simulink model "power_brushlessDCmotor_moog2328_control_scheme"  (R2022a)
settings: Solver=ode4  StartTime=0  StopTime=2  FixedStep=Ts  MaxStep=1e-6  RelTol=1e-6  AbsTol=1e-6  EnableMultiTasking=on
PreLoadFcn:
  | assignin('base','Ts',[5e-6])
values from neighbouring files (symbols this model uses):
  F = 49.387e-4*2/1000    (= 9.8774e-06)    [power_brushlessDCmotor_moog2328_control_scheme.m]
  J = 465.8e-7    (= 4.658e-05)    [power_brushlessDCmotor_moog2328_control_scheme.m]
  La = 0.17e-3    (= 0.00017)    [power_brushlessDCmotor_moog2328_control_scheme.m]
  Lb = 0.17e-3    (= 0.00017)    [power_brushlessDCmotor_moog2328_control_scheme.m]
  Lc = 0.17e-3    (= 0.00017)    [power_brushlessDCmotor_moog2328_control_scheme.m]
  N = 297.5    [power_brushlessDCmotor_moog2328_control_scheme.m]
  p = 4    [power_brushlessDCmotor_moog2328_control_scheme.m]
  Ra = 0.1    [power_brushlessDCmotor_moog2328_control_scheme.m]
  Rb = 0.1    [power_brushlessDCmotor_moog2328_control_scheme.m]
  Rc = 0.1    [power_brushlessDCmotor_moog2328_control_scheme.m]
  trap = sin((pi-Flat/180*pi)/2)    [power_brushlessDCmotor_moog2328_control_scheme.m]
  Ts = 5e-5    (= 5e-05)    [power_brushlessDCmotor_moog2328_control_scheme.m]
undefined symbols (not defined in the file or in its folder): DiscIntNeverNeededParam, find_system, sgn
libraries: simulink x7, spsDiodeLib x6, spsMosfetLib x6, spsCurrentMeasurementLib x4, spsVoltageMeasurementLib x4, spsParallelRLCBranchLib x3, spsGroundLib x3, spsControlledVoltageSourceLib x3, spsSeriesRLCBranchLib x3, simulink_extras x3, spsDCVoltageSourceLib x1, spspowerguiLib x1
Description:
  | This demonstration illustrates use of the BLDC in a closed-loop
  | speed and voltage control on a 1 kW, 3000 rpm industrial motor
settings Model: Creator=Olivier Tremblay  LastModifiedBy=marin
settings SolverCC: AutoScaleAbsTol=off  AlgebraicLoopSolver=TrustRegion
settings DataIOCC: LimitDataPoints=on  SaveFormat=Array  SignalLoggingSaveFormat=ModelDataLogs  ReturnWorkspaceOutputs=off  SignalLoggingName=sigsOut
settings OptimizationCC: ExpressionDepthLimit=2147483647  InitFltsAndDblsToZero=on  LifeSpan=inf
settings DebuggingCC: SaveWithParameterizedLinksMsg=none  UnderspecifiedInitializationDetection=Classic  MergeDetectMultiDrivingBlocksExec=none  SignalResolutionControl=TryResolveAllWithWarning  MultiTaskDSMMsg=warning  MultiTaskCondExecSysMsg=none  SigSpecEnsureSampleTimeMsg=none  FcnCallInpInsideContextMsg=warning  UnconnectedInputMsg=warning  UnconnectedOutputMsg=warning  UnconnectedLineMsg=warning  StateNameClashWarn=warning  SFUnexpectedBacktrackingDiag=warning  SFNoUnconditionalDefaultTransitionDiag=warning  SFExecutionAtInitializationDiag=none  SFMachineParentedDataDiag=warning  ArithmeticOperatorsInVariantConditions=warning
settings HardwareCC: ProdBitPerPointer=32  ProdBitPerSizeT=32  ProdBitPerPtrDiffT=32  ProdLargestAtomicFloat=None  ProdIntDivRoundTo=Undefined  ProdEndianess=Unspecified  ProdWordSize=32  ProdHWDeviceType=32-bit Generic  TargetUnknown=on
settings ModelReferenceCC: PropagateSignalLabelsOutOfModel=off
settings SFSimCC: SimUseLocalCustomCode=off  CustomCodeUndefinedFunction=UseInterfaceOnly
settings RTWCC: RTWUseLocalCustomCode=off  DLArmComputeVersion=19.05
settings CodeAppCC: StateflowObjectComments=on
settings GRTTargetCC: TargetFcnLib=ansi_tfl_tmw.mat  TargetLangStandard=C89/C90 (ANSI)  CombineOutputUpdateFcns=off  GRTInterface=on
settings ConfigComp: CovMetricSettings=dw  CovSaveCumulativeToWorkspaceVar=on  CovSaveSingleToWorkspaceVar=on  CovExternalEMLEnable=off
settings SimscapeCC: SimscapeNormalizeSystem=off

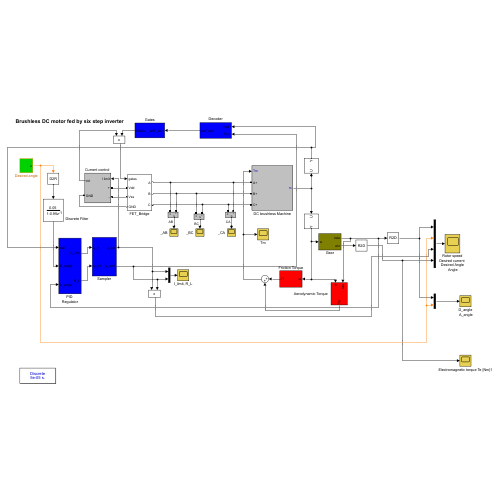
[thumbnail: Simulink's stored preview of the top-level diagram]
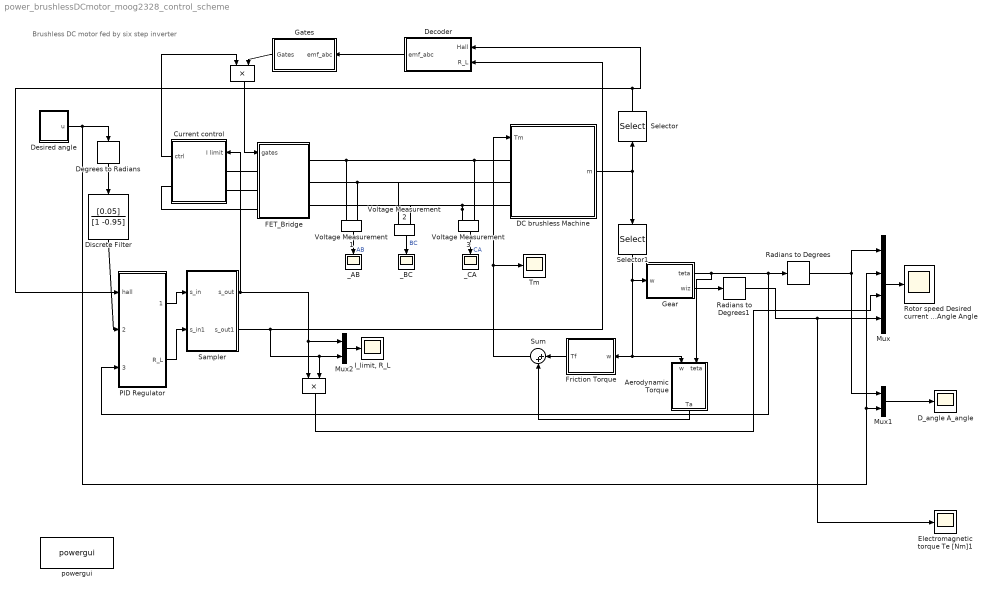
== system power_brushlessDCmotor_moog2328_control_scheme ==
  note: Brushless DC motor fed by six step inverter
  " " : Product  RndMeth=Zero
  " " : Product  RndMeth=Zero
  " Discrete Filter" : DiscreteFilter  Numerator=[0.05]  Denominator=[1 -0.95]  SampleTime=Ts
  " Current control " : Subsystem  mask(Current control){R=0.02, R1=0.01, C=4700e-6, V1=14.31/100, V=28}
      mask prompts: R "Resistance R [ohm]"; R1 "Resistance R1 [ohm]"; C "Capacitance C [F]"; V1 "Control voltage [V]"; V "DC source [V]"
  "Aerodynamic Torque " : Subsystem  mask(Aerodynamic Torque and friction){Ta=100, G=N, eta=0.7, Tgv=0, Tgf=0}
      mask prompts: Ta "Aerodinamic Torque [Nm]"; G "Gear coeficient"; eta "Eficiency"; Tgv "Fg viscous friction"; Tgf "Kgf columb friction"
  DC brushless Machine : Subsystem  AncestorBlock=powerlib/Machines/DC Machine  LoadFcn=find_system(gcs,'FollowLinks', 'on', 'LookUnderMasks', 'all');
      settings: OpenFcn=power_openblockproxy();
  D_angle A_angle : Scope
  Decoder : Subsystem  mask(Decoder){}
      mask help:
      | Hal
      | 	to	emf_abc
      | R or L
  Degrees to Radians : simulink_extras/Transformations/Degrees to Radians
  "Desired angle " : Subsystem  mask(Deaired angle){Fo=1, f=2.5, of=6, ch=1, an=-1}
      mask prompts: Fo "Desired angle [deg]"; f "Freqency [Hz]"; of "ofs"; ch "1 for sin(x), -1 for square(x)"; an "1 for angle meas. -1 for simul."
      mask init:
      | Fid=Fo
  Electromagnetic torque Te [Nm]1 : Scope
  FET_Bridge : Subsystem
  Friction Torque : Subsystem  mask(Friction Torque){Tf=0.303*0.05}
      mask prompts: Tf "Friction Torque [Nm]"
  Gates : Subsystem  mask(Gates){}
      mask help: Convert emf_abc in to signal for gates
  Gear : Subsystem  mask(Gear){}
      mask help: Integration and gear reduction
  "I_limit, R_L" : Scope
  Mux : Mux
  Mux1 : Mux  Inputs=2
  Mux2 : Mux  Inputs=2
  PID Regulator : Subsystem  mask(PID Regulator){KI=27.0082733381866, KP=1.97984715541991*65, KD=0.0105535523473669*35, Ao=10, Inom=14.31, Boost=1}
      mask prompts: KI "Integral gain"; KP "Proportional gain"; KD "Differential gain"; Ao "Ao gain"; Inom "Nominal current [A]"
  Radians to Degrees : simulink_extras/Transformations/Radians to Degrees
  Radians to Degrees1 : simulink_extras/Transformations/Radians to Degrees
  Rotor speed Desired current Desired Angle Angle : Scope
  Sampler : Subsystem
  Selector : Selector  InputPortWidth=12  IndexOptions=Index vector (dialog)  Indices=[7:9]  OutputSizes=1
  Selector1 : Selector  InputPortWidth=12  IndexOptions=Index vector (dialog)  Indices=10  OutputSizes=1
  Sum : Sum  Inputs=|++
  Tm : Scope
  Voltage Measurement1 : spsVoltageMeasurementLib/Voltage Measurement  PhasorSimulation=off  OutputType=Complex  PSBequivalent=0
  Voltage Measurement2 : spsVoltageMeasurementLib/Voltage Measurement  PhasorSimulation=off  OutputType=Complex  PSBequivalent=0
  Voltage Measurement3 : spsVoltageMeasurementLib/Voltage Measurement  PhasorSimulation=off  OutputType=Complex  PSBequivalent=0
  _AB : Scope
  _BC : Scope
  _CA : Scope
  powergui : spspowerguiLib/powergui  Priority=2  SimulationMode=Discrete  SampleTime=5e-5  frequency=60  Iterations=50  frequencyindice=0  Pbase=100e6  ErrMax=1e-4  UnitsV=kV  UnitsW=MW  buscounter=0  FunctionMessages=off  echomessages=off  EnableUseOfTLC=off  CurrentSourceSwitches=off  DisableSnubberDevices=off  DisableRonSwitches=off  DisableVfSwitches=off  DisplayEquations=off  AutomaticDiscreteSolvers=off  SolverType=Tustin  Interpol=off  ExternalGateDelay=off  methode=off  Ts=0  x0status=blocks  SPID=off  SwTol=0  HookPort=off  NonlinearTolerance=1e-4  nMaxIteration=100  ContinueOnMaxIteration=off  RestoreLinks=warning  ResistiveCurrentMeasurement=off  Frange=[0:2:500]  Ylog=off  Xlog=on  ShowGrid=off  save=off  variable=ZData  structure=0  ZoomFFT=on  StartTime=0.0  cycles=1  DisplayStyle=1  fundamental=60  FreqAxis=off  MaxFrequency=1000  frequencyindicesteady=1  RmsSteady=1  display=off
  wires:
  DC brushless Machine/1(m) -> Selector1/1, Selector/1
  Gear/1(teta) -> "Aerodynamic Torque "/2(teta), PID Regulator/3(A_angle), Radians to Degrees/1
  Sum/1 -> Tm/1, DC brushless Machine/1(Tm)
  Degrees to Radians/1 -> " Discrete Filter"/1
  Voltage Measurement1/1 -> _AB/1  "AB"
  Decoder/1(emf_abc) -> Gates/1("emf_abc ")
  "Desired angle "/1(u) -> Degrees to Radians/1, Mux1/2, Mux/2
  Mux/1 -> Rotor speed Desired current Desired Angle Angle/1
  Radians to Degrees/1 -> Mux1/1, Mux/1
  Gates/1(Gates) -> " "/2
  Voltage Measurement2/1 -> _BC/1  "BC"
  Voltage Measurement3/1 -> _CA/1  "CA"
  Friction Torque/1(Tf) -> Sum/1
  "Aerodynamic Torque "/1(Ta) -> Sum/2
  Mux1/1 -> D_angle A_angle/1
  Mux2/1 -> "I_limit, R_L"/1
  " "/1 -> Mux/3
  " Current control "/1(ctrl) -> " "/1
  " "/1 -> FET_Bridge/1(gates)
  " Discrete Filter"/1 -> PID Regulator/2(D_angle)
  Sampler/2(s_out1) -> Decoder/2(R_L), Mux2/2, " "/2
  Sampler/1(s_out) -> " Current control "/1(I limit), Mux2/1, " "/1
  PID Regulator/1(I_Limit) -> Sampler/1(s_in)
  PID Regulator/2(R_L) -> Sampler/2(s_in1)
  Gear/2(wiz) -> Radians to Degrees1/1
  Radians to Degrees1/1 -> Electromagnetic torque Te [Nm]1/1, Mux/4
  Selector/1 -> PID Regulator/1(hall), Decoder/1("Hall ")
  Selector1/1 -> Gear/1(w), Friction Torque/1(w), "Aerodynamic Torque "/1(w)
  connections:
  DC brushless Machine/LConn2 -- Voltage Measurement2/LConn1 -- FET_Bridge/RConn2 -- Voltage Measurement1/LConn2
  Voltage Measurement3/LConn1 -- DC brushless Machine/LConn3 -- FET_Bridge/RConn3 -- Voltage Measurement2/LConn2
  FET_Bridge/LConn1 -- " Current control "/LConn1
  " Current control "/LConn2 -- FET_Bridge/LConn2
  " Current control "/RConn1 -- FET_Bridge/LConn3
  FET_Bridge/RConn1 -- DC brushless Machine/LConn1 -- Voltage Measurement3/LConn2 -- Voltage Measurement1/LConn1

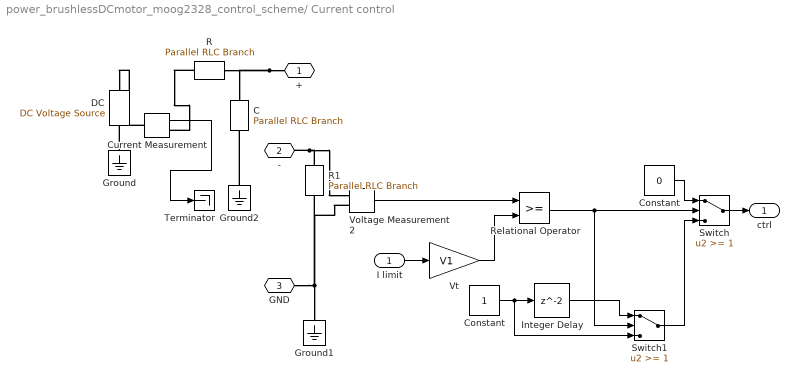
== system power_brushlessDCmotor_moog2328_control_scheme/ Current control  ==
  I limit : Inport
  " C" : spsParallelRLCBranchLib/Parallel RLC Branch  LConnTagsString=a  RConnTagsString=__new0  BranchType=C  Resistance=0.02  Inductance=1e-3  SetiL0=off  InitialCurrent=0  Capacitance=C  Setx0=off  InitialVoltage=0  Measurements=None
  " R" : spsParallelRLCBranchLib/Parallel RLC Branch  LConnTagsString=a  RConnTagsString=__new0  BranchType=R  Resistance=R  Inductance=1e-3  SetiL0=off  InitialCurrent=0  Capacitance=1e-6  Setx0=off  InitialVoltage=0  Measurements=None
  " R1" : spsParallelRLCBranchLib/Parallel RLC Branch  LConnTagsString=a  RConnTagsString=__new0  BranchType=R  Resistance=R1  Inductance=1e-3  SetiL0=off  InitialCurrent=0  Capacitance=1e-6  Setx0=off  InitialVoltage=0  Measurements=None
  Constant : Constant  Value=0  SampleTime=Ts
  "Constant " : Constant  SampleTime=Ts
  Current Measurement : spsCurrentMeasurementLib/Current Measurement  PhasorSimulation=off  OutputType=Complex  PSBequivalent=0
  "DC " : spsDCVoltageSourceLib/DC Voltage Source  Amplitude=V  Measurements=None
  Ground : spsGroundLib/Ground  LConnTagsString=a
  Ground1 : spsGroundLib/Ground  LConnTagsString=a
  Ground2 : spsGroundLib/Ground  LConnTagsString=a
  Integer Delay : Delay  InitialCondition=0  SampleTime=Ts
  Relational Operator : RelationalOperator  OutDataTypeStr=boolean  SampleTime=Ts  InputSameDT=off
  Switch : Switch  Threshold=1  SampleTime=Ts  SaturateOnIntegerOverflow=off  InputSameDT=off
  Switch1 : Switch  Threshold=1  SampleTime=Ts  SaturateOnIntegerOverflow=off  InputSameDT=off
  Terminator : Terminator
  Voltage Measurement2 : spsVoltageMeasurementLib/Voltage Measurement  PhasorSimulation=off  OutputType=Complex  PSBequivalent=0
  Vt : Gain  Gain=V1  SampleTime=Ts
  + : PMIOPort  Side=Left
  - : PMIOPort  Port=2  Side=Left
  GND : PMIOPort  Port=3  Side=Right
  ctrl : Outport
  wires:
  I limit/1 -> Vt/1
  Voltage Measurement2/1 -> Relational Operator/1
  Vt/1 -> Relational Operator/2
  Relational Operator/1 -> Switch/2, Switch1/2
  Constant/1 -> Switch/1
  Switch/1 -> ctrl/1
  "Constant "/1 -> Integer Delay/1, Switch1/3
  Integer Delay/1 -> Switch1/1
  Switch1/1 -> Switch/3
  Current Measurement/1 -> Terminator/1
  connections:
  -/RConn1 -- Voltage Measurement2/LConn1 -- " R1"/LConn1
  " R1"/RConn1 -- Voltage Measurement2/LConn2 -- Ground1/LConn1 -- GND/RConn1
  +/RConn1 -- " R"/RConn1 -- " C"/LConn1
  Ground2/LConn1 -- " C"/RConn1
  Current Measurement/LConn1 -- "DC "/RConn1
  Ground/LConn1 -- "DC "/LConn1
  " R"/LConn1 -- Current Measurement/RConn1

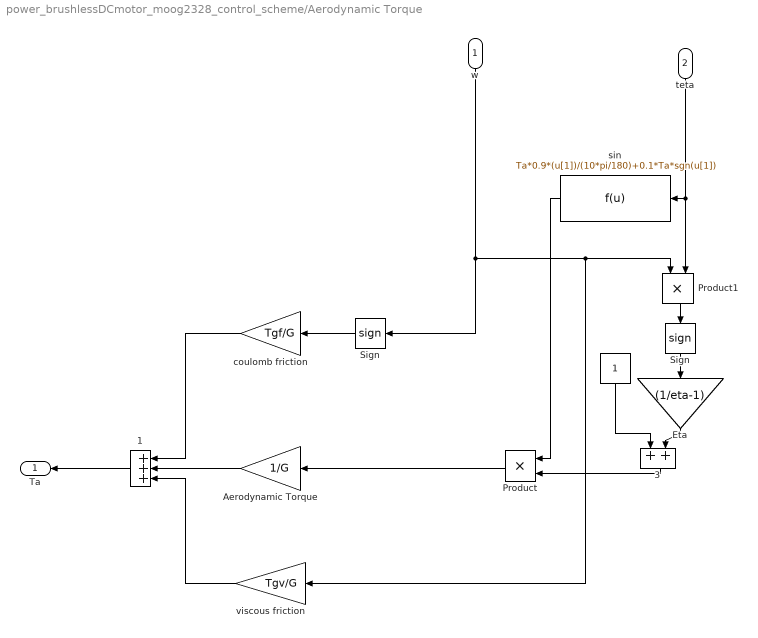
== system power_brushlessDCmotor_moog2328_control_scheme/Aerodynamic Torque  ==
  w : Inport
  teta : Inport  Port=2
  " " : Constant  SampleTime=Ts
  "    1" : Sum  Inputs=+++  InputSameDT=on  SaturateOnIntegerOverflow=on  SampleTime=Ts  OutDataTypeStr=Inherit: Same as first input
  "    3" : Sum  InputSameDT=on  SaturateOnIntegerOverflow=on  SampleTime=Ts  OutDataTypeStr=Inherit: Same as first input
  Aerodynamic Torque : Gain  Gain=1/G  SaturateOnIntegerOverflow=on  SampleTime=Ts  OutDataTypeStr=Inherit: Same as input  ParamDataTypeStr=Inherit: Same as input
  Eta : Gain  Gain=(1/eta-1)  SaturateOnIntegerOverflow=on  SampleTime=Ts  OutDataTypeStr=Inherit: Same as input  ParamDataTypeStr=Inherit: Same as input
  Product : Product  RndMeth=Zero  SampleTime=Ts
  Product1 : Product  RndMeth=Zero  SampleTime=Ts
  Sign : Signum  SampleTime=Ts
  "Sign " : Signum  SampleTime=Ts
  coulomb friction : Gain  Gain=Tgf/G  SaturateOnIntegerOverflow=on  SampleTime=Ts  OutDataTypeStr=Inherit: Same as input  ParamDataTypeStr=Inherit: Same as input
  sin : Fcn  Expr=Ta*0.9*(u[1])/(10*pi/180)+0.1*Ta*sgn(u[1])  SampleTime=Ts
  viscous friction : Gain  Gain=Tgv/G  SaturateOnIntegerOverflow=on  SampleTime=Ts  OutDataTypeStr=Inherit: Same as input  ParamDataTypeStr=Inherit: Same as input
  Ta : Outport
  wires:
  Product1/1 -> Sign/1
  sin/1 -> Product/1
  Sign/1 -> Eta/1
  " "/1 -> "    3"/1
  Eta/1 -> "    3"/2
  w/1 -> Product1/1, viscous friction/1, "Sign "/1
  teta/1 -> sin/1, Product1/2
  Product/1 -> Aerodynamic Torque/1
  "    1"/1 -> Ta/1
  Aerodynamic Torque/1 -> "    1"/2
  viscous friction/1 -> "    1"/3
  "Sign "/1 -> coulomb friction/1
  coulomb friction/1 -> "    1"/1
  "    3"/1 -> Product/2

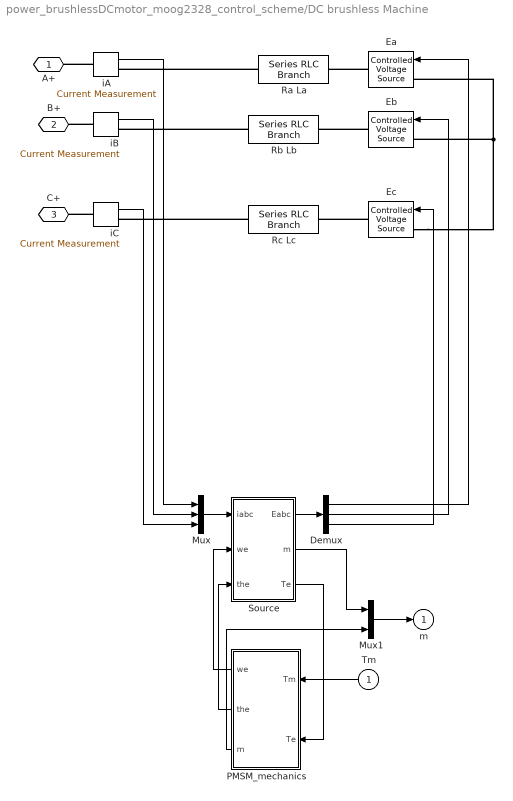
== system power_brushlessDCmotor_moog2328_control_scheme/DC brushless Machine ==
  Tm : Inport
  Demux : Demux  Outputs=3
  Ea : spsControlledVoltageSourceLib/Controlled Voltage Source  Description=source block  Initialize=on  Source_Type=AC  Amplitude=0  Phase=0  Frequency=0  Measurements=None
  Eb : spsControlledVoltageSourceLib/Controlled Voltage Source  Description=source block  Initialize=on  Source_Type=AC  Amplitude=0  Phase=0  Frequency=0  Measurements=None
  Ec : spsControlledVoltageSourceLib/Controlled Voltage Source  Description=source block  Initialize=on  Source_Type=AC  Amplitude=0  Phase=0  Frequency=0  Measurements=None
  Mux : Mux  Inputs=3
  Mux1 : Mux  Inputs=2
  PMSM_mechanics : Subsystem  AncestorBlock=powerlib_models/Discrete/PM_trapezoidal_mechanics
  Ra La : spsSeriesRLCBranchLib/Series RLC Branch  LConnTagsString=__new0  RConnTagsString=__new0  BranchType=RL  Resistance=Ra  Inductance=La  SetiL0=off  InitialCurrent=0  Capacitance=inf  Setx0=off  InitialVoltage=0  Measurements=None
  Rb Lb : spsSeriesRLCBranchLib/Series RLC Branch  LConnTagsString=__new0  RConnTagsString=__new0  BranchType=RL  Resistance=Rb  Inductance=Lb  SetiL0=off  InitialCurrent=0  Capacitance=inf  Setx0=off  InitialVoltage=0  Measurements=None
  Rc Lc : spsSeriesRLCBranchLib/Series RLC Branch  LConnTagsString=__new0  RConnTagsString=__new0  BranchType=RL  Resistance=Rc  Inductance=Lc  SetiL0=off  InitialCurrent=0  Capacitance=inf  Setx0=off  InitialVoltage=0  Measurements=None
  Source : Subsystem  AncestorBlock=powerlib_models/Discrete/PM_trapezoidal
  iA : spsCurrentMeasurementLib/Current Measurement  PhasorSimulation=off  OutputType=Magnitude  PSBequivalent=0
  iB : spsCurrentMeasurementLib/Current Measurement  PhasorSimulation=off  OutputType=Magnitude  PSBequivalent=0
  iC : spsCurrentMeasurementLib/Current Measurement  PhasorSimulation=off  OutputType=Magnitude  PSBequivalent=0
  A+ : PMIOPort  Side=Left
  B+ : PMIOPort  Port=2  Side=Left
  C+ : PMIOPort  Port=3  Side=Left
  m : Outport  InitialOutput=0
  wires:
  PMSM_mechanics/1(we) -> Source/2(we)
  PMSM_mechanics/2(the) -> Source/3(the)
  PMSM_mechanics/3(m) -> Mux1/2
  Tm/1 -> PMSM_mechanics/1(Tm)
  Source/2(m) -> Mux1/1
  Source/3(Te) -> PMSM_mechanics/2(Te)
  Mux1/1 -> m/1
  Mux/1 -> Source/1(iabc)
  iA/1 -> Mux/1
  iB/1 -> Mux/2
  iC/1 -> Mux/3
  Source/1(Eabc) -> Demux/1
  Demux/1 -> Ea/1
  Demux/2 -> Eb/1
  Demux/3 -> Ec/1
  connections:
  Eb/LConn1 -- Ec/LConn1 -- Ea/LConn1
  iA/LConn1 -- A+/RConn1
  Ea/RConn1 -- Ra La/RConn1
  Ra La/LConn1 -- iA/RConn1
  iB/LConn1 -- B+/RConn1
  Eb/RConn1 -- Rb Lb/RConn1
  Rb Lb/LConn1 -- iB/RConn1
  iC/LConn1 -- C+/RConn1
  Ec/RConn1 -- Rc Lc/RConn1
  Rc Lc/LConn1 -- iC/RConn1

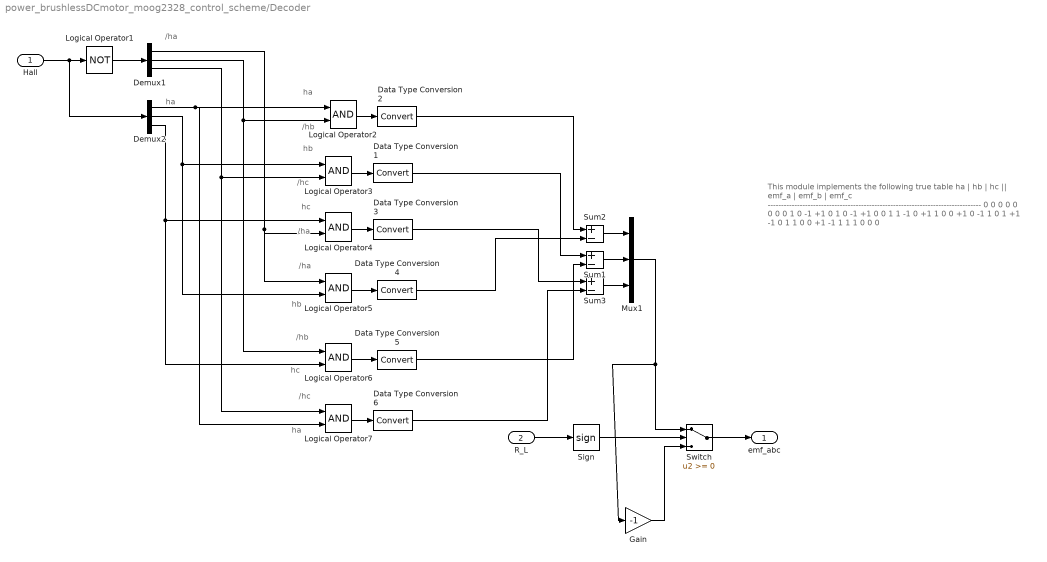
== system power_brushlessDCmotor_moog2328_control_scheme/Decoder ==
  note: /ha
  note: ha
  note: ha
  note: /hb
  note: hb
  note: /hc
  note: hc
  note: /ha
  note: /ha
  note: hb
  note: /hb
  note: hc
  note: /hc
  note: ha
  note: This module implements the following true table
      |
      |    ha   |   hb   |   hc   ||   emf_a   |   emf_b   |   emf_c
      |     --------------------------------------------------------------------------------
      | 0          0         0          0               0               0
      | 0          0         1          0               -1              +1
      | 0          1         0          -1              +1                0
      | 0          1         1          -1               0               +1
      | 1          0         0         +1               0               -1
      | 1          0         1         +1              -1                0
      | 1          1         0          0              +1               -1
      | 1          1         1          0               0                0
  "Hall " : Inport
  R_L : Inport  Port=2
  Data Type Conversion{1..6} (6 alike) : DataTypeConversion  SaturateOnIntegerOverflow=off  RndMeth=Floor
  Demux1 : Demux  Outputs=3
  Demux2 : Demux  Outputs=3
  Gain : Gain  Gain=-1
  Logical Operator1 : Logic  Operator=NOT  AllPortsSameDT=off  OutDataTypeStr=boolean
  Logical Operator{2..7} (6 alike) : Logic  AllPortsSameDT=off  OutDataTypeStr=boolean
  Mux1 : Mux  Inputs=3
  Sign : Signum
  Sum1 : Sum  Inputs=+-  OutDataTypeStr=double
  Sum2 : Sum  Inputs=+-  OutDataTypeStr=double
  Sum3 : Sum  Inputs=+-  OutDataTypeStr=double
  Switch : Switch  SaturateOnIntegerOverflow=off  InputSameDT=off
  emf_abc : Outport
  wires:
  "Hall "/1 -> Logical Operator1/1, Demux2/1
  Logical Operator1/1 -> Demux1/1
  Demux2/3 -> Logical Operator4/1, Logical Operator6/2
  Demux2/2 -> Logical Operator3/1, Logical Operator5/2
  Demux2/1 -> Logical Operator2/1, Logical Operator7/2
  Demux1/3 -> Logical Operator3/2, Logical Operator7/1
  Demux1/2 -> Logical Operator2/2, Logical Operator6/1
  Demux1/1 -> Logical Operator4/2, Logical Operator5/1
  Logical Operator2/1 -> Data Type Conversion2/1
  Sum2/1 -> Mux1/1
  Sum1/1 -> Mux1/2
  Sum3/1 -> Mux1/3
  Logical Operator3/1 -> Data Type Conversion1/1
  Logical Operator4/1 -> Data Type Conversion3/1
  Logical Operator5/1 -> Data Type Conversion4/1
  Logical Operator6/1 -> Data Type Conversion5/1
  Logical Operator7/1 -> Data Type Conversion6/1
  R_L/1 -> Sign/1
  Sign/1 -> Switch/2
  Mux1/1 -> Switch/1, Gain/1
  Switch/1 -> emf_abc/1
  Data Type Conversion2/1 -> Sum2/1
  Data Type Conversion4/1 -> Sum2/2
  Data Type Conversion1/1 -> Sum1/1
  Data Type Conversion5/1 -> Sum1/2
  Data Type Conversion3/1 -> Sum3/1
  Data Type Conversion6/1 -> Sum3/2
  Gain/1 -> Switch/3

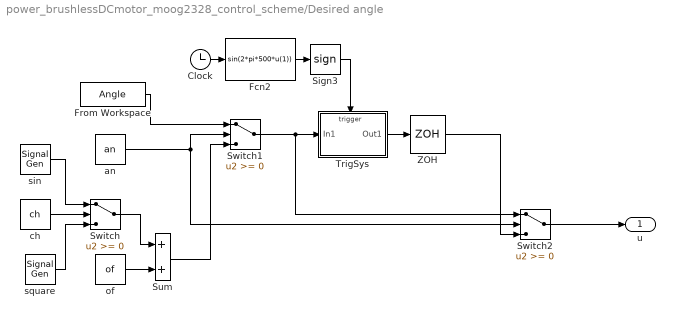
== system power_brushlessDCmotor_moog2328_control_scheme/Desired angle  ==
  Clock : Clock
  Fcn2 : Fcn  Expr=sin(2*pi*500*u(1))
  From Workspace : FromWorkspace  VariableName=Angle  SampleTime=Ts
  Sign3 : Signum
  Sum : Sum  SaturateOnIntegerOverflow=on
  Switch : Switch  SampleTime=Ts  SaturateOnIntegerOverflow=off  InputSameDT=off
  Switch1 : Switch  SampleTime=Ts  SaturateOnIntegerOverflow=off  InputSameDT=off
  Switch2 : Switch  SampleTime=Ts  SaturateOnIntegerOverflow=off  InputSameDT=off
  TrigSys : Subsystem  TreatAsAtomicUnit=on
  ZOH : ZeroOrderHold  SampleTime=Ts
  an : Constant  Value=an
  ch : Constant  Value=ch
  of : Constant  Value=of
  sin : SignalGenerator  Amplitude=Fid  Frequency=f
  square : SignalGenerator  WaveForm=square  Amplitude=-Fid  Frequency=f
  u : Outport
  wires:
  of/1 -> Sum/2
  Sum/1 -> Switch1/3
  From Workspace/1 -> Switch1/1
  TrigSys/1(Out1) -> ZOH/1
  Switch1/1 -> TrigSys/1(In1), Switch2/1
  Clock/1 -> Fcn2/1
  Fcn2/1 -> Sign3/1
  Sign3/1 -> TrigSys/Trigger
  Switch2/1 -> u/1
  sin/1 -> Switch/1
  square/1 -> Switch/3
  Switch/1 -> Sum/1
  ch/1 -> Switch/2
  an/1 -> Switch1/2, Switch2/2
  ZOH/1 -> Switch2/3

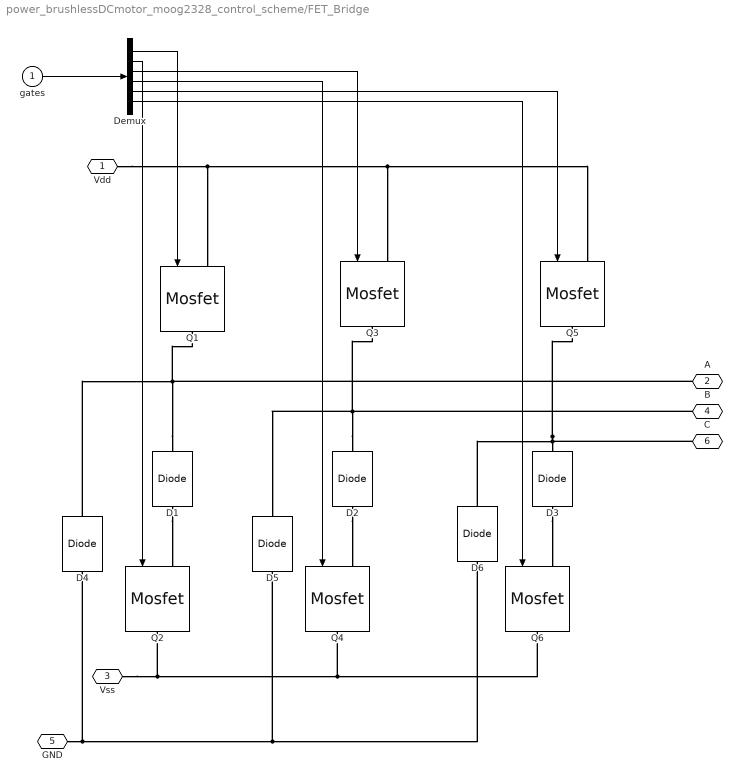
== system power_brushlessDCmotor_moog2328_control_scheme/FET_Bridge ==
  gates : Inport
  D{1..6} (6 alike) : spsDiodeLib/Diode  Ron=0.05  Lon=0  Vf=0.5  IC=0  UseSnubber=off  Rs=5000  Cs=1e-6  Measurements=off
  Demux : Demux  Outputs=6
  Q{1..6} (6 alike) : spsMosfetLib/Mosfet  Ron=0.05  Lon=0  Rd=0.05  Vfd=0.5  IC=0  Rs=5000  Cs=1e-6  Measurements=off
  Vdd : PMIOPort  Side=Left
  A : PMIOPort  Port=2  Side=Right
  Vss : PMIOPort  Port=3  Side=Left
  B : PMIOPort  Port=4  Side=Right
  GND : PMIOPort  Port=5  Side=Left
  C : PMIOPort  Port=6  Side=Right
  wires:
  gates/1 -> Demux/1
  Demux/1 -> Q1/1
  Demux/2 -> Q2/1
  Demux/3 -> Q3/1
  Demux/4 -> Q4/1
  Demux/5 -> Q5/1
  Demux/6 -> Q6/1
  connections:
  Q4/RConn1 -- Vss/RConn1 -- Q2/RConn1 -- Q6/RConn1
  Vdd/RConn1 -- Q1/LConn1 -- Q5/LConn1 -- Q3/LConn1
  D6/LConn1 -- D4/LConn1 -- GND/RConn1 -- D5/LConn1
  D3/LConn1 -- D6/RConn1 -- C/RConn1 -- Q5/RConn1
  D2/LConn1 -- Q3/RConn1 -- D5/RConn1 -- B/RConn1
  D1/LConn1 -- D4/RConn1 -- Q1/RConn1 -- A/RConn1
  D3/RConn1 -- Q6/LConn1
  D2/RConn1 -- Q4/LConn1
  D1/RConn1 -- Q2/LConn1

== system power_brushlessDCmotor_moog2328_control_scheme/Friction Torque ==
  w : Inport
  Friction Torque : Gain  Gain=Tf  SaturateOnIntegerOverflow=on  OutDataTypeStr=Inherit: Same as input  ParamDataTypeStr=Inherit: Same as input
  Sign : Signum
  Tf : Outport
  wires:
  Sign/1 -> Friction Torque/1
  w/1 -> Sign/1
  Friction Torque/1 -> Tf/1

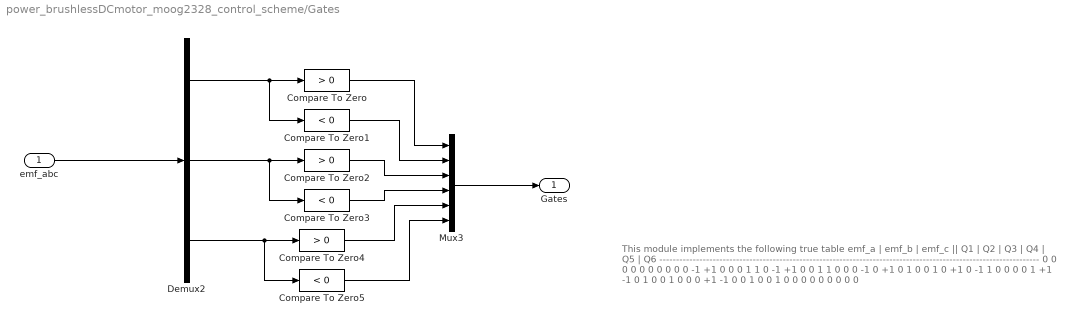
== system power_brushlessDCmotor_moog2328_control_scheme/Gates ==
  note: This module implements the following true table
      |
      |    emf_a   |   emf_b   |   emf_c   ||   Q1   |   Q2   |   Q3   |   Q4   |   Q5   |   Q6
      |     ------------------------------------------------------------------------------------------------------------------
      |       0              0                0            0          0          0           0        0        0
      |       0               -1              +1          0          0          0           1        1        0
      |     -1              +1                0          0          1          1           0        0        0
      |     -1               0               +1          0          1         0           0        1        0
      |    +1               0                -1          1          0          0           0        0        1
      |    +1              -1                0           1          0          0           1        0        0
      |      0              +1               -1           0          0          1           0        0        1
      |     0              0                0             0          0          0           0        0        0
  "emf_abc " : Inport
  Compare To Zero : simulink/Logic and Bit Operations/Compare To Zero  relop=>  OutDataTypeStr=boolean  ZeroCross=off
  Compare To Zero1 : simulink/Logic and Bit Operations/Compare To Zero  relop=<  OutDataTypeStr=boolean  ZeroCross=off
  Compare To Zero2 : simulink/Logic and Bit Operations/Compare To Zero  relop=>  OutDataTypeStr=boolean  ZeroCross=off
  Compare To Zero3 : simulink/Logic and Bit Operations/Compare To Zero  relop=<  OutDataTypeStr=boolean  ZeroCross=off
  Compare To Zero4 : simulink/Logic and Bit Operations/Compare To Zero  relop=>  OutDataTypeStr=boolean  ZeroCross=off
  Compare To Zero5 : simulink/Logic and Bit Operations/Compare To Zero  relop=<  OutDataTypeStr=boolean  ZeroCross=off
  Demux2 : Demux  Outputs=3
  Mux3 : Mux  Inputs=6
  Gates : Outport
  wires:
  "emf_abc "/1 -> Demux2/1
  Demux2/1 -> Compare To Zero/1, Compare To Zero1/1
  Demux2/2 -> Compare To Zero2/1, Compare To Zero3/1
  Demux2/3 -> Compare To Zero4/1, Compare To Zero5/1
  Compare To Zero/1 -> Mux3/1
  Compare To Zero1/1 -> Mux3/2
  Compare To Zero2/1 -> Mux3/3
  Compare To Zero3/1 -> Mux3/4
  Compare To Zero4/1 -> Mux3/5
  Compare To Zero5/1 -> Mux3/6
  Mux3/1 -> Gates/1

== system power_brushlessDCmotor_moog2328_control_scheme/Gear ==
  w : Inport
  Discrete-Time Integrator : DiscreteIntegrator  SampleTime=Ts  ICPrevOutput=DiscIntNeverNeededParam  ICPrevScaledInput=DiscIntNeverNeededParam
  Fcn3 : Fcn  Expr=u[1]/N  SampleTime=Ts
  teta : Outport
  wiz : Outport  Port=2
  wires:
  w/1 -> Fcn3/1
  Discrete-Time Integrator/1 -> teta/1
  Fcn3/1 -> Discrete-Time Integrator/1, wiz/1

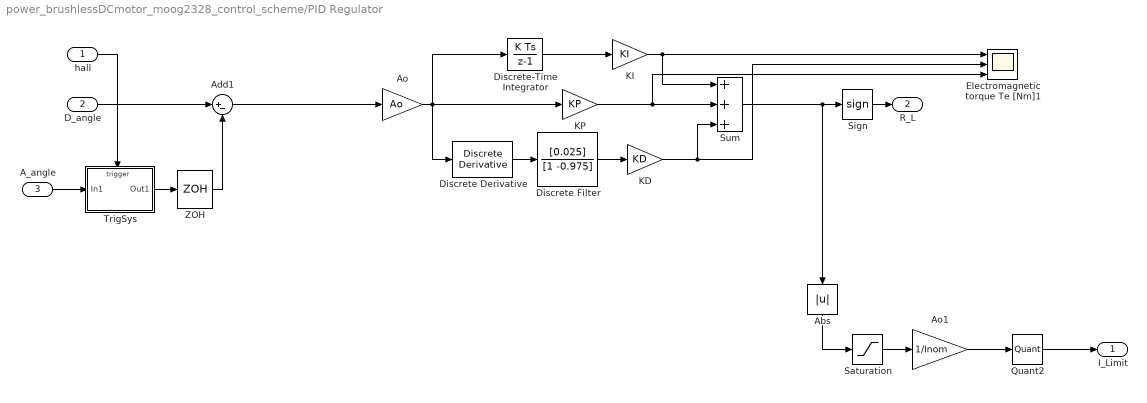
== system power_brushlessDCmotor_moog2328_control_scheme/PID Regulator ==
  hall : Inport
  D_angle : Inport  Port=2
  A_angle : Inport  Port=3
  "Abs " : Abs
  Add1 : Sum  Inputs=|+-
  Ao : Gain  Gain=Ao  SaturateOnIntegerOverflow=on  SampleTime=Ts  OutDataTypeStr=Inherit: Same as input  ParamDataTypeStr=Inherit: Same as input
  Ao1 : Gain  Gain=1/Inom  SaturateOnIntegerOverflow=on  SampleTime=Ts  OutDataTypeStr=Inherit: Same as input  ParamDataTypeStr=Inherit: Same as input
  Discrete Derivative : simulink/Discrete/Discrete Derivative  gainval=1.0  ICPrevScaledInput=0.0  OutMin=[]  OutMax=[]  OutDataType=sfix(16)  OutScaling=2^-10  DoSatur=off
      link override Diff: OutDataTypeMode=Inherit via back propagation
  Discrete Filter : DiscreteFilter  Numerator=[0.025]  Denominator=[1 -0.975]  SampleTime=Ts
  Discrete-Time Integrator : DiscreteIntegrator  SampleTime=Ts  ICPrevOutput=DiscIntNeverNeededParam  ICPrevScaledInput=DiscIntNeverNeededParam
  Electromagnetic torque Te [Nm]1 : Scope  NumInputPorts=3
  KD : Gain  Gain=KD  SaturateOnIntegerOverflow=on  SampleTime=Ts  OutDataTypeStr=Inherit: Same as input  ParamDataTypeStr=Inherit: Same as input
  KI : Gain  Gain=KI  SaturateOnIntegerOverflow=on  SampleTime=Ts  OutDataTypeStr=Inherit: Same as input  ParamDataTypeStr=Inherit: Same as input
  KP : Gain  Gain=KP  SaturateOnIntegerOverflow=on  SampleTime=Ts  OutDataTypeStr=Inherit: Same as input  ParamDataTypeStr=Inherit: Same as input
  Quant2 : Quantizer  QuantizationInterval=Boost/20
  Saturation : Saturate  UpperLimit=Inom*Boost  LowerLimit=-Inom*Boost
  "Sign " : Signum  SampleTime=Ts
  Sum : Sum  Inputs=+++  SaturateOnIntegerOverflow=on  SampleTime=Ts
  TrigSys : Subsystem  TreatAsAtomicUnit=on
  ZOH : ZeroOrderHold  SampleTime=Ts
  I_Limit : Outport
  R_L : Outport  Port=2
  wires:
  Sum/1 -> "Sign "/1, "Abs "/1
  Discrete-Time Integrator/1 -> KI/1
  KP/1 -> Sum/2, Electromagnetic torque Te [Nm]1/3
  KD/1 -> Sum/3, Electromagnetic torque Te [Nm]1/2
  "Sign "/1 -> R_L/1
  TrigSys/1(Out1) -> ZOH/1
  Discrete Derivative/1 -> Discrete Filter/1
  D_angle/1 -> Add1/1
  A_angle/1 -> TrigSys/1(In1)
  ZOH/1 -> Add1/2
  hall/1 -> TrigSys/Trigger
  Discrete Filter/1 -> KD/1
  Ao/1 -> KP/1, Discrete Derivative/1, Discrete-Time Integrator/1
  KI/1 -> Sum/1, Electromagnetic torque Te [Nm]1/1
  Add1/1 -> Ao/1
  "Abs "/1 -> Saturation/1
  Saturation/1 -> Ao1/1
  Ao1/1 -> Quant2/1
  Quant2/1 -> I_Limit/1

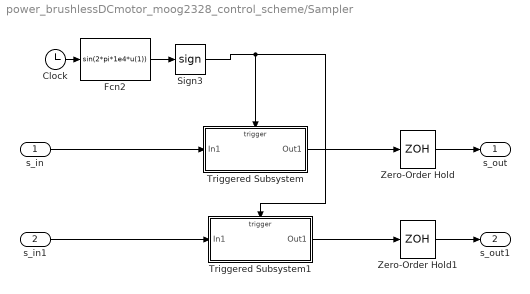
== system power_brushlessDCmotor_moog2328_control_scheme/Sampler ==
  s_in : Inport
  s_in1 : Inport  Port=2
  Clock : Clock
  Fcn2 : Fcn  Expr=sin(2*pi*1e4*u(1))  SampleTime=Ts
  Sign3 : Signum
  Triggered Subsystem : Subsystem  TreatAsAtomicUnit=on
  Triggered Subsystem1 : Subsystem  TreatAsAtomicUnit=on
  Zero-Order Hold : ZeroOrderHold  SampleTime=-1
  Zero-Order Hold1 : ZeroOrderHold  SampleTime=-1
  s_out : Outport
  s_out1 : Outport  Port=2
  wires:
  Sign3/1 -> Triggered Subsystem/Trigger, Triggered Subsystem1/Trigger
  s_in/1 -> Triggered Subsystem/1(In1)
  Zero-Order Hold/1 -> s_out/1
  Triggered Subsystem/1(Out1) -> Zero-Order Hold/1
  s_in1/1 -> Triggered Subsystem1/1(In1)
  Triggered Subsystem1/1(Out1) -> Zero-Order Hold1/1
  Zero-Order Hold1/1 -> s_out1/1
  Clock/1 -> Fcn2/1
  Fcn2/1 -> Sign3/1

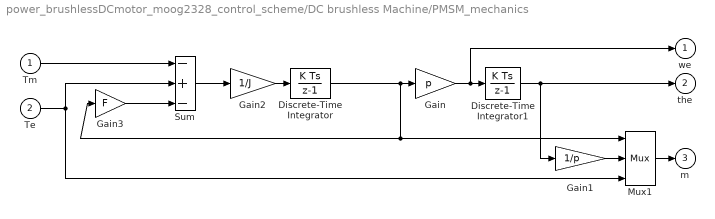
== system power_brushlessDCmotor_moog2328_control_scheme/DC brushless Machine/PMSM_mechanics ==
  Tm : Inport
  Te : Inport  Port=2
  Discrete-Time Integrator : DiscreteIntegrator  SampleTime=Ts  ICPrevOutput=DiscIntNeverNeededParam  ICPrevScaledInput=DiscIntNeverNeededParam
  Discrete-Time Integrator1 : DiscreteIntegrator  SampleTime=Ts  ICPrevOutput=DiscIntNeverNeededParam  ICPrevScaledInput=DiscIntNeverNeededParam
  Gain : Gain  Gain=p  SaturateOnIntegerOverflow=on  SampleTime=Ts  OutDataTypeStr=Inherit: Same as input  ParamDataTypeStr=Inherit: Same as input
  Gain1 : Gain  Gain=1/p  SaturateOnIntegerOverflow=on  SampleTime=Ts  OutDataTypeStr=Inherit: Same as input  ParamDataTypeStr=Inherit: Same as input
  Gain2 : Gain  Gain=1/J  SaturateOnIntegerOverflow=on  SampleTime=Ts  OutDataTypeStr=Inherit: Same as input  ParamDataTypeStr=Inherit: Same as input
  Gain3 : Gain  Gain=F  SaturateOnIntegerOverflow=on  SampleTime=Ts  OutDataTypeStr=Inherit: Same as input  ParamDataTypeStr=Inherit: Same as input
  Mux1 : Mux  Inputs=3
  Sum : Sum  Inputs=-+-  InputSameDT=on  SaturateOnIntegerOverflow=on  SampleTime=Ts  OutDataTypeStr=Inherit: Same as first input
  we : Outport  InitialOutput=0
  the : Outport  Port=2  InitialOutput=0
  m : Outport  Port=3  InitialOutput=0
  wires:
  Te/1 -> Sum/2, Mux1/3
  Gain3/1 -> Sum/3
  Mux1/1 -> m/1
  Tm/1 -> Sum/1
  Sum/1 -> Gain2/1
  Gain2/1 -> Discrete-Time Integrator/1
  Discrete-Time Integrator/1 -> Gain/1, Mux1/1, Gain3/1
  Discrete-Time Integrator1/1 -> the/1, Gain1/1
  Gain1/1 -> Mux1/2
  Gain/1 -> we/1, Discrete-Time Integrator1/1

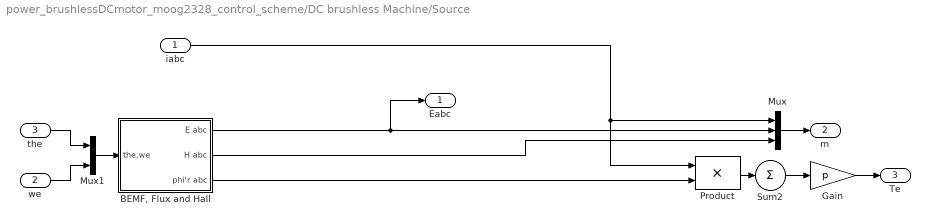
== system power_brushlessDCmotor_moog2328_control_scheme/DC brushless Machine/Source ==
  iabc : Inport
  we : Inport  Port=2
  the : Inport  Port=3
  "BEMF, Flux and Hall" : Subsystem
  Gain : Gain  Gain=p  SaturateOnIntegerOverflow=on  SampleTime=Ts  OutDataTypeStr=Inherit: Same as input  ParamDataTypeStr=Inherit: Same as input
  Mux : Mux  Inputs=3
  Mux1 : Mux  Inputs=2
  Product : Product  SaturateOnIntegerOverflow=on  SampleTime=Ts  OutDataTypeStr=Inherit: Same as first input
  Sum2 : Sum  Inputs=+  SaturateOnIntegerOverflow=on  SampleTime=Ts
  Eabc : Outport  InitialOutput=0
  m : Outport  Port=2  InitialOutput=0
  Te : Outport  Port=3  InitialOutput=0
  wires:
  Mux/1 -> m/1
  "BEMF, Flux and Hall"/2(H abc) -> Mux/3
  iabc/1 -> Mux/1, Product/1
  Sum2/1 -> Gain/1
  "BEMF, Flux and Hall"/3(phi'r abc) -> Product/2
  Mux1/1 -> "BEMF, Flux and Hall"/1(the,we)
  Product/1 -> Sum2/1
  "BEMF, Flux and Hall"/1(E abc) -> Mux/2, Eabc/1
  we/1 -> Mux1/2
  the/1 -> Mux1/1
  Gain/1 -> Te/1

== system power_brushlessDCmotor_moog2328_control_scheme/Desired angle /TrigSys ==
  In1 : Inport
  Trigger : TriggerPort  VariantControl=(inherit)
  Out1 : Outport
  wires:
  In1/1 -> Out1/1

== system power_brushlessDCmotor_moog2328_control_scheme/PID Regulator/TrigSys ==
  In1 : Inport
  Trigger : TriggerPort  TriggerType=either  VariantControl=(inherit)
  Out1 : Outport
  wires:
  In1/1 -> Out1/1

== system power_brushlessDCmotor_moog2328_control_scheme/Sampler/Triggered Subsystem ==
  In1 : Inport
  Trigger : TriggerPort  TriggerType=either  VariantControl=(inherit)
  Out1 : Outport
  wires:
  In1/1 -> Out1/1

== system power_brushlessDCmotor_moog2328_control_scheme/Sampler/Triggered Subsystem1 ==
  In1 : Inport
  Trigger : TriggerPort  TriggerType=either  VariantControl=(inherit)
  Out1 : Outport
  wires:
  In1/1 -> Out1/1

== system power_brushlessDCmotor_moog2328_control_scheme/DC brushless Machine/Source/BEMF, Flux and Hall ==
  the,we : Inport
  Mux4 : Mux  Inputs=3
  Mux6 : Mux  Inputs=3
  Mux7 : Mux  Inputs=3
  Phase a : Subsystem
  Phase b : Subsystem
  Phase c : Subsystem
  E abc : Outport
  H abc : Outport  Port=2
  phi'r abc : Outport  Port=3
  wires:
  Mux6/1 -> H abc/1
  Mux7/1 -> phi'r abc/1
  Mux4/1 -> E abc/1
  Phase c/1(phi'r) -> Mux7/3
  Phase b/1(phi'r) -> Mux7/2
  Phase a/1(phi'r) -> Mux7/1
  Phase c/3(H) -> Mux6/3
  Phase b/3(H) -> Mux6/2
  Phase a/3(H) -> Mux6/1
  Phase c/2(E) -> Mux4/3
  Phase b/2(E) -> Mux4/2
  Phase a/2(E) -> Mux4/1
  the,we/1 -> Phase c/1(the,we), Phase b/1(the,we), Phase a/1(the,we)

== system power_brushlessDCmotor_moog2328_control_scheme/DC brushless Machine/Source/BEMF, Flux and Hall/Phase a ==
  note: Phi' r
  the,we : Inport
  Demux : Demux  Outputs=2
      settings: DisplayOption=none
  Fcn : Fcn  Expr=cos(u[1])  SampleTime=Ts
  Gain4 : Gain  Gain=Flux/trap  SaturateOnIntegerOverflow=on  SampleTime=Ts  OutDataTypeStr=Inherit: Same as input  ParamDataTypeStr=Inherit: Same as input
  Hall sensor : Subsystem
  Product1 : Product  SaturateOnIntegerOverflow=on  SampleTime=Ts  OutDataTypeStr=Inherit: Same as first input
  Saturation : Saturate  UpperLimit=trap  LowerLimit=-trap  SampleTime=Ts
  phi'r : Outport
  E : Outport  Port=2
  H : Outport  Port=3
  wires:
  Hall sensor/1(Hall) -> H/1
  Gain4/1 -> Product1/1, phi'r/1
  Product1/1 -> E/1
  the,we/1 -> Demux/1
  Demux/2 -> Product1/2
  Fcn/1 -> Saturation/1
  Demux/1 -> Fcn/1, Hall sensor/1(the)
  Saturation/1 -> Gain4/1

== system power_brushlessDCmotor_moog2328_control_scheme/DC brushless Machine/Source/BEMF, Flux and Hall/Phase b ==
  note: Phi' r
  the,we : Inport
  Demux : Demux  Outputs=2
      settings: DisplayOption=none
  Fcn : Fcn  Expr=cos(u[1]-2*pi/3)  SampleTime=Ts
  Gain4 : Gain  Gain=Flux/trap  SaturateOnIntegerOverflow=on  SampleTime=Ts  OutDataTypeStr=Inherit: Same as input  ParamDataTypeStr=Inherit: Same as input
  Hall sensor : Subsystem
  Product1 : Product  SaturateOnIntegerOverflow=on  SampleTime=Ts  OutDataTypeStr=Inherit: Same as first input
  Saturation : Saturate  UpperLimit=trap  LowerLimit=-trap  SampleTime=Ts
  phi'r : Outport
  E : Outport  Port=2
  H : Outport  Port=3
  wires:
  Saturation/1 -> Gain4/1
  Demux/1 -> Fcn/1, Hall sensor/1(the)
  Fcn/1 -> Saturation/1
  Demux/2 -> Product1/2
  the,we/1 -> Demux/1
  Product1/1 -> E/1
  Gain4/1 -> phi'r/1, Product1/1
  Hall sensor/1(Hall) -> H/1

== system power_brushlessDCmotor_moog2328_control_scheme/DC brushless Machine/Source/BEMF, Flux and Hall/Phase c ==
  note: Phi' r
  the,we : Inport
  Demux : Demux  Outputs=2
      settings: DisplayOption=none
  Fcn : Fcn  Expr=cos(u[1]+2*pi/3)  SampleTime=Ts
  Gain4 : Gain  Gain=Flux/trap  SaturateOnIntegerOverflow=on  SampleTime=Ts  OutDataTypeStr=Inherit: Same as input  ParamDataTypeStr=Inherit: Same as input
  Hall sensor : Subsystem
  Product1 : Product  SaturateOnIntegerOverflow=on  SampleTime=Ts  OutDataTypeStr=Inherit: Same as first input
  Saturation : Saturate  UpperLimit=trap  LowerLimit=-trap  SampleTime=Ts
  phi'r : Outport
  E : Outport  Port=2
  H : Outport  Port=3
  wires:
  Gain4/1 -> Product1/1, phi'r/1
  Product1/1 -> E/1
  the,we/1 -> Demux/1
  Demux/2 -> Product1/2
  Fcn/1 -> Saturation/1
  Demux/1 -> Fcn/1, Hall sensor/1(the)
  Saturation/1 -> Gain4/1
  Hall sensor/1(Hall) -> H/1

== system power_brushlessDCmotor_moog2328_control_scheme/DC brushless Machine/Source/BEMF, Flux and Hall/Phase a/Hall sensor ==
  the : Inport
  Constant : Constant  SampleTime=Ts
  Fcn : Fcn  Expr=sin(u[1]+pi/3)  SampleTime=Ts
  Gain : Gain  Gain=0.5  SampleTime=Ts
  Sign : Signum  SampleTime=Ts
  Sum : Sum  SampleTime=Ts
  Hall : Outport
  wires:
  the/1 -> Fcn/1
  Fcn/1 -> Sign/1
  Sign/1 -> Sum/1
  Constant/1 -> Sum/2
  Sum/1 -> Gain/1
  Gain/1 -> Hall/1

== system power_brushlessDCmotor_moog2328_control_scheme/DC brushless Machine/Source/BEMF, Flux and Hall/Phase b/Hall sensor ==
  the : Inport
  Constant : Constant  SampleTime=Ts
  Fcn1 : Fcn  Expr=sin(u[1]-pi/3)  SampleTime=Ts
  Gain : Gain  Gain=0.5  SampleTime=Ts
  Sign : Signum  SampleTime=Ts
  Sum : Sum  SampleTime=Ts
  Hall : Outport
  wires:
  the/1 -> Fcn1/1
  Fcn1/1 -> Sign/1
  Sign/1 -> Sum/1
  Constant/1 -> Sum/2
  Sum/1 -> Gain/1
  Gain/1 -> Hall/1

== system power_brushlessDCmotor_moog2328_control_scheme/DC brushless Machine/Source/BEMF, Flux and Hall/Phase c/Hall sensor ==
  the : Inport
  Constant : Constant  SampleTime=Ts
  Fcn1 : Fcn  Expr=sin(u[1]+pi)  SampleTime=Ts
  Gain : Gain  Gain=0.5  SampleTime=Ts
  Sign : Signum  SampleTime=Ts
  Sum : Sum  SampleTime=Ts
  Hall : Outport
  wires:
  the/1 -> Fcn1/1
  Fcn1/1 -> Sign/1
  Sign/1 -> Sum/1
  Constant/1 -> Sum/2
  Sum/1 -> Gain/1
  Gain/1 -> Hall/1
